simulink model "lin_spaceship_v5"  (Simulink 7.8)
settings: Solver=ode45  StartTime=0  StopTime=100  FixedStep=dt_sim  RelTol=1e-6
undefined symbols (not defined in the file): JB, X0
libraries: vrlib x1
settings Model: Creator=vickTJ  LastModifiedBy=Dan  BufferReuse=off
settings SolverCC: MaxConsecutiveMinStep=3
settings DataIOCC: ExternalInput=a  InitialState=[]  LimitDataPoints=off  MaxDataPoints=5000  SaveState=on  SignalLogging=off  DSMLogging=off  StateSaveName=stout
settings OptimizationCC: InlineParams=on  BufferReuse=off
settings DebuggingCC: SolverPrmCheckMsg=none  FcnCallInpInsideContextMsg=Use local settings  UnconnectedInputMsg=none  UnconnectedOutputMsg=none  InitInArrayFormatMsg=none  SFInvalidInputDataAccessInChartInitDiag=none

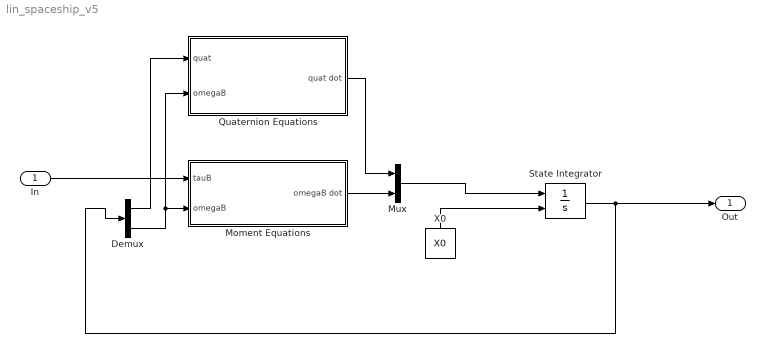
== system lin_spaceship_v5 ==
  In : Inport
  Demux : Demux  Outputs=2
  Moment Equations : Subsystem
  Mux : Mux  Inputs=2
  Quaternion Equations : Subsystem
  State Integrator : Integrator  InitialConditionSource=external
  X0 : Constant  Value=X0
  Out : Outport
  wires:
  X0/1 -> State Integrator/2
  State Integrator/1 -> Demux/1, Out/1
  Demux/1 -> Quaternion Equations/1(quat)
  Demux/2 -> Quaternion Equations/2(omegaB), Moment Equations/2(omegaB)
  Quaternion Equations/1(quat dot) -> Mux/1
  Moment Equations/1(omegaB dot) -> Mux/2
  Mux/1 -> State Integrator/1
  In/1 -> Moment Equations/1(tauB)

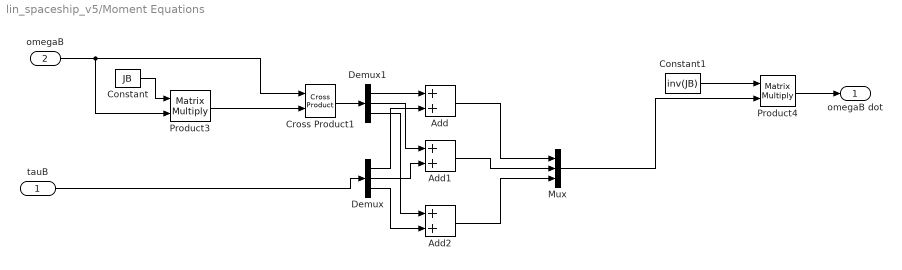
== system lin_spaceship_v5/Moment Equations ==
  tauB : Inport  OutDataTypeStr=double
  omegaB : Inport  Port=2
  Add : Sum
  Add1 : Sum
  Add2 : Sum
  Constant : Constant  Value=JB
  Constant1 : Constant  Value=inv(JB)
  Cross Product1 : vrlib/Utilities/Cross Product
  Demux : Demux  Outputs=3
  Demux1 : Demux  Outputs=3
  Mux : Mux  Inputs=3
  Product3 : Product  Multiplication=Matrix(*)  RndMeth=Zero
  Product4 : Product  Multiplication=Matrix(*)  RndMeth=Zero
  omegaB dot : Outport
  wires:
  Product4/1 -> omegaB dot/1
  Constant/1 -> Product3/1
  omegaB/1 -> Product3/2, Cross Product1/1
  Product3/1 -> Cross Product1/2
  Constant1/1 -> Product4/1
  tauB/1 -> Demux/1
  Cross Product1/1 -> Demux1/1
  Demux1/1 -> Add/1
  Demux/1 -> Add/2
  Demux1/2 -> Add1/1
  Demux/2 -> Add1/2
  Demux1/3 -> Add2/1
  Demux/3 -> Add2/2
  Add/1 -> Mux/1
  Add1/1 -> Mux/2
  Add2/1 -> Mux/3
  Mux/1 -> Product4/2

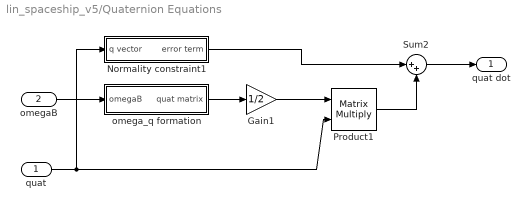
== system lin_spaceship_v5/Quaternion Equations ==
  quat : Inport
  omegaB : Inport  Port=2
  Gain1 : Gain  Gain=1/2
  Normality constraint1 : Subsystem
  Product1 : Product  Multiplication=Matrix(*)  RndMeth=Zero
  Sum2 : Sum  Inputs=|++
  omega_q formation : Subsystem
  quat dot : Outport
  wires:
  quat/1 -> Product1/2, Normality constraint1/1(q vector)
  Gain1/1 -> Product1/1
  omega_q formation/1(quat matrix) -> Gain1/1
  omegaB/1 -> omega_q formation/1(omegaB)
  Product1/1 -> Sum2/2
  Sum2/1 -> quat dot/1
  Normality constraint1/1(error term) -> Sum2/1

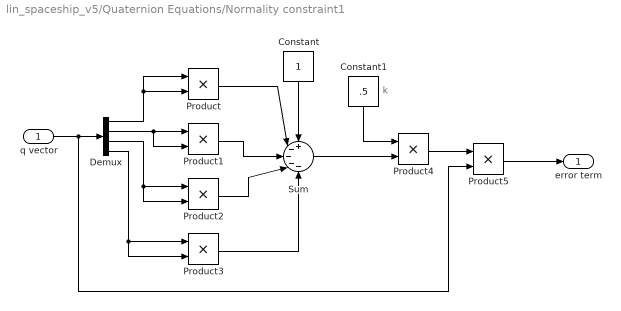
== system lin_spaceship_v5/Quaternion Equations/Normality constraint1 ==
  note: k
  q vector : Inport
  Constant : Constant
  Constant1 : Constant  Value=.5
  Demux : Demux
  Product{,1..5} (6 alike) : Product  RndMeth=Zero
  Sum : Sum  Inputs=+----
  error term : Outport
  wires:
  Product5/1 -> error term/1
  q vector/1 -> Product5/2, Demux/1
  Product4/1 -> Product5/1
  Sum/1 -> Product4/2
  Constant1/1 -> Product4/1
  Product3/1 -> Sum/5
  Product2/1 -> Sum/4
  Product1/1 -> Sum/3
  Product/1 -> Sum/2
  Constant/1 -> Sum/1
  Demux/4 -> Product3/1, Product3/2
  Demux/3 -> Product2/2, Product2/1
  Demux/2 -> Product1/2, Product1/1
  Demux/1 -> Product/1, Product/2

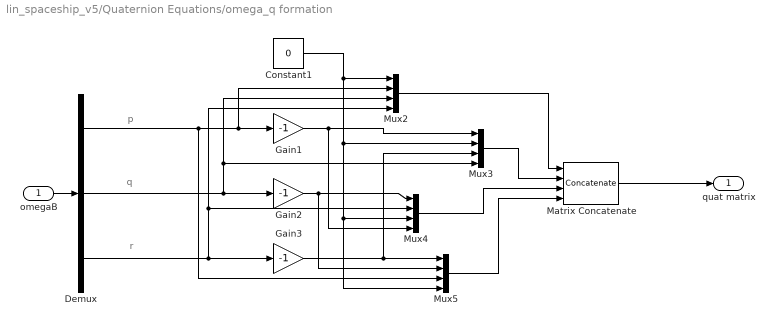
== system lin_spaceship_v5/Quaternion Equations/omega_q formation ==
  note: r
  note: q
  note: p
  omegaB : Inport
  Constant1 : Constant  Value=0
  Demux : Demux  Outputs=3
  Gain1 : Gain  Gain=-1
  Gain2 : Gain  Gain=-1
  Gain3 : Gain  Gain=-1
  Matrix Concatenate : Concatenate  NumInputs=4  Mode=Multidimensional array  ConcatenateDimension=2
  Mux{2..5} (4 alike) : Mux
  quat matrix : Outport
  wires:
  omegaB/1 -> Demux/1
  Matrix Concatenate/1 -> quat matrix/1
  Mux5/1 -> Matrix Concatenate/4
  Mux4/1 -> Matrix Concatenate/3
  Mux3/1 -> Matrix Concatenate/2
  Mux2/1 -> Matrix Concatenate/1
  Constant1/1 -> Mux2/1, Mux3/2, Mux4/3, Mux5/4
  Demux/1 -> Gain1/1, Mux2/2, Mux5/3
  Demux/2 -> Gain2/1, Mux2/3, Mux3/4
  Demux/3 -> Gain3/1, Mux2/4, Mux4/2
  Gain1/1 -> Mux3/1, Mux4/4
  Gain3/1 -> Mux3/3, Mux5/1
  Gain2/1 -> Mux4/1, Mux5/2
